simulink model "HevP1OptimalController"  (R2023b)
settings: configuration reference "VehicleFixed10ms" (kept outside this file)
model workspace (MAT data in the model file):
  N_P0 = 1
undefined symbols (not defined in the file): CtrlBcuTrlrBrkGain, CtrlVcuHevPxChrgLmtBpt, CtrlVcuHevPxRegenBrkCutOff, CtrlVcuHevPxSocBpt, PlntBrkActrBoreFrnt, PlntBrkFrntBias, PlntBrkKinFricCffFrnt, PlntBrkNumPadsFrnt, PlntBrkPadMeanRadiusFrnt, PlntBrkPrsFctr, PlntBrkRearBias, PlntDCDCEff, PlntDiffrntlEff, PlntDiffrntlRatio, PlntEM1EffTbl, PlntEM1Spd, PlntEM1Trq, PlntEngAccPwrTbl, PlntEngAccSpdBpt, PlntEngBrkTrqSpdBpt, PlntTransEffSpdBpt, PlntTransEffTbl, PlntTransEffTempBpt, PlntTransEffTrqBpt, PlntTransGearNumVect, PlntTransGearRatioVect, PlntWhlLdRadius
libraries: simulink x2, autolibhevctrlr x1, autolibhevctrlrcommon x1
settings Model: DataDictionary=VirtualVehicleTemplate.sldd  ModifiedByFormat=The MathWorks, Inc.  Creator=The MathWorks, Inc.  LastModifiedBy=The MathWorks, Inc.
settings ConfigSetRef: SourceName=VehicleFixed10ms

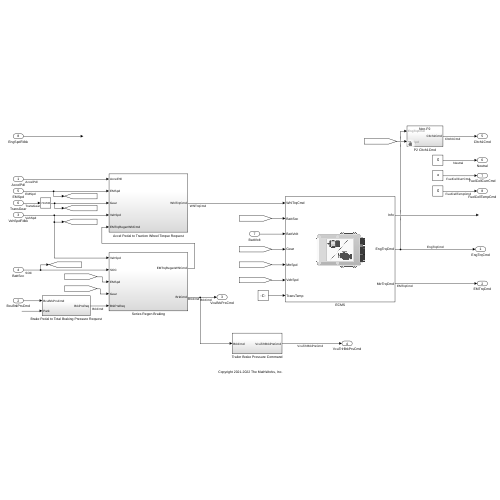
[thumbnail: Simulink's stored preview of the top-level diagram]
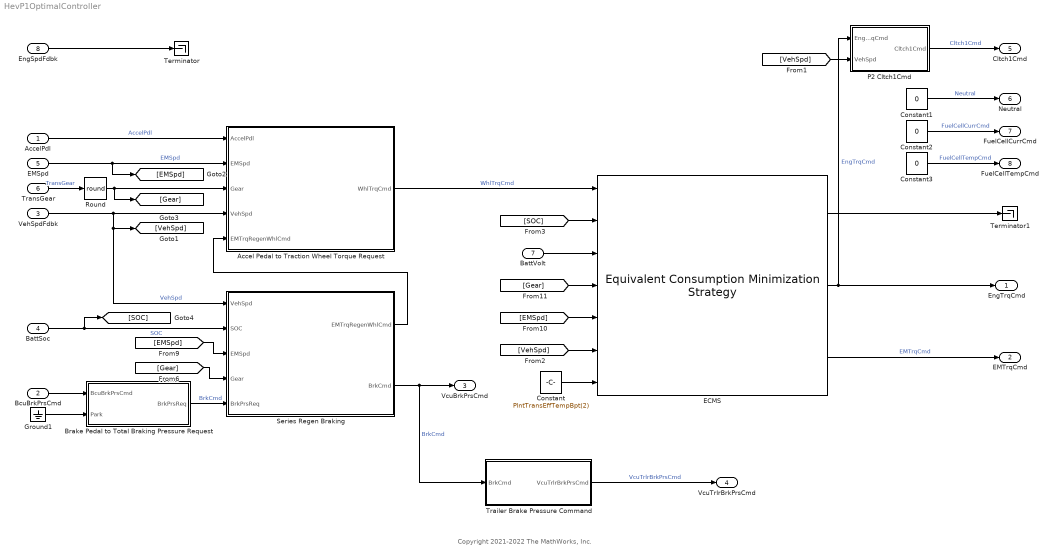
== system HevP1OptimalController ==
  note: Copyright 2021-2022 The MathWorks, Inc.
  AccelPdl : Inport  OutDataTypeStr=double  PortDimensions=1
  "   BcuBrkPrsCmd   " : Inport  Port=2  OutDataTypeStr=double  PortDimensions=4
  VehSpdFdbk : Inport  Port=3  OutDataTypeStr=double  PortDimensions=1
  BattSoc : Inport  Port=4  OutDataTypeStr=double  PortDimensions=1
  EMSpd : Inport  Port=5  OutDataTypeStr=double  PortDimensions=1
  TransGear : Inport  Port=6  OutDataTypeStr=double  PortDimensions=1
  BattVolt : Inport  Port=7  OutDataTypeStr=double  PortDimensions=1
  EngSpdFdbk : Inport  Port=8  OutDataTypeStr=double  PortDimensions=1
  Accel Pedal to Traction Wheel Torque Request : Subsystem  InitFcn=[~]=autosharedicon('autolibinternalvvblock',gcb,0);
  Brake Pedal to Total Braking Pressure Request : Subsystem
  Constant : Constant  Value=PlntTransEffTempBpt(2)
  Constant1 : Constant  Value=0  SampleTime=-1
  Constant2 : Constant  Value=0  SampleTime=-1
  Constant3 : Constant  Value=0  SampleTime=-1
  ECMS : autolibhevctrlr/Equivalent Consumption Minimization Strategy  HevMtrLoc=P1  EcmsMethod=Non-adaptive  N_diff=PlntDiffrntlRatio  eta_diff=PlntDiffrntlEff  N_diff_P4=PlntDiffrntl2Ratio  Re=PlntWhlLdRadius  TransEffFactors=Gear, input torque, input speed, and temperature  G_trans=PlntTransGearNumVect  N_trans=PlntTransGearRatioVect  Trq_trans_bpts=PlntTransEffTrqBpt  omega_trans_bpts=PlntTransEffSpdBpt  Temp_trans_bpts=PlntTransEffTempBpt  eta_trans=PlntTransEffVect  eta_trans_tbl=PlntTransEffTbl  f_tbrake_n_bpt=PlntEngBrkTrqSpdBpt  f_tbrake_t_bpt=PlntEngBrkTrqBpt  f_tbrake=PlntEngBrkTrqMap  f_tbrake_min=CtrlVcuHevPxEngTrqMin  f_fuel=PlntEngFuelFlwMap  HEVEngTrq_min=CtrlVcuHevPxHEVEngTrqMin  LHV=PlntEngLhv  AccPwrTbl=[0 0]  AccSpdBpts=[300 750]  N_idle=CtrlEcuNidle  SOC_bpt=CtrlVcuHevPxSocBpt  ChrgLmt=CtrlVcuHevPxChrgLmtBpt  DischrgLmt=CtrlVcuHevPxDischrgLmtBpt  BattCurrMax=CtrlVcuHevPxBattCurrMax  eta_dcdc=PlntDCDCEff/100  BattChrgPwrMax=CtrlVcuHevPxBattChrgPwrMax  BattDischrgPwrMax=CtrlVcuHevPxBattDischrgPwrMax  MtrEffiMethod=Positive speed and full torque range  f_tmtr_max=PlntEM1Trq  f_mtr_w_bpt=PlntEM1Spd*30/pi  f_mtr_t_bpt=PlntEM1TrqEff  f_mtr_eta=PlntEM1EffTbl/100  Ngrid=CtrlVcuHevPxNgrid  N_P0=PlntDiffrntlP0Ratio  ECMS_s=CtrlVcuHevP1ECMSs  a=CtrlVcuHevPxPnltyFctr  ECMS_Kp=CtrlVcuHevPxAdaptECMSKpGain  ECMS_Ki=CtrlVcuHevPxAdaptECMSKiGain  PenaltyFctr=CtrlVcuHevPxPenaltyFctr  SOCTrgt=CtrlVcuHevPxSOCTrgt  SOCmin=CtrlVcuHevPxSOCmin  SOCmax=CtrlVcuHevPxSOCmax
  Ground1 : Ground
  P2 Cltch1Cmd : Subsystem  Variant=on  VariantControlMode=label  VariantControl=1  LabelModeActiveChoice=0
  Round : Rounding  Operator=round
  Series Regen Braking : Subsystem  InitFcn=[~]=autosharedicon('autolibinternalvvblock',gcb,0);  VariantControl=0
  Terminator : Terminator
  Terminator1 : Terminator
  Trailer Brake Pressure Command : Subsystem
  EngTrqCmd : Outport  OutDataTypeStr=double  Unit=N*m  PortDimensions=1  VectorParamsAs1DForOutWhenUnconnected=off
  EMTrqCmd : Outport  Port=2  OutDataTypeStr=double  Unit=N*m  PortDimensions=1  VectorParamsAs1DForOutWhenUnconnected=off
  VcuBrkPrsCmd : Outport  Port=3  OutDataTypeStr=double  PortDimensions=4  VectorParamsAs1DForOutWhenUnconnected=off
  VcuTrlrBrkPrsCmd : Outport  Port=4  PortDimensions=6  VectorParamsAs1DForOutWhenUnconnected=off
  Cltch1Cmd : Outport  Port=5  OutDataTypeStr=double  PortDimensions=1  VectorParamsAs1DForOutWhenUnconnected=off
  Neutral : Outport  Port=6  OutDataTypeStr=double  PortDimensions=1  VectorParamsAs1DForOutWhenUnconnected=off
  FuelCellCurrCmd : Outport  Port=7  OutDataTypeStr=double  PortDimensions=1
  FuelCellTempCmd : Outport  Port=8  OutDataTypeStr=double  PortDimensions=1
  wires:
  AccelPdl/1 -> Accel Pedal to Traction Wheel Torque Request/1(AccelPdl)  "AccelPdl"
  "   BcuBrkPrsCmd   "/1 -> Brake Pedal to Total Braking Pressure Request/1(BcuBrkPrsCmd)
  VehSpdFdbk/1 -> Series Regen Braking/1(VehSpd), [VehSpd], Accel Pedal to Traction Wheel Torque Request/4(VehSpd)  "VehSpd"
  [SOC] -> ECMS/2
  EMSpd/1 -> [EMSpd], Accel Pedal to Traction Wheel Torque Request/2(EMSpd)  "EMSpd"
  Accel Pedal to Traction Wheel Torque Request/1(WhlTrqCmd) -> ECMS/1  "WhlTrqCmd"
  Ground1/1 -> Brake Pedal to Total Braking Pressure Request/2(Park)
  TransGear/1 -> Round/1  "TransGear"
  Brake Pedal to Total Braking Pressure Request/1(BrkPrsReq) -> Series Regen Braking/5("BrkPrsReq ")  "BrkCmd"
  Series Regen Braking/1(" EMTrqRegenWhlCmd") -> Accel Pedal to Traction Wheel Torque Request/5(EMTrqRegenWhlCmd)
  [EMSpd] -> Series Regen Braking/3(EMSpd)
  [Gear] -> Series Regen Braking/4(Gear)
  Constant1/1 -> Neutral/1  "Neutral"
  [VehSpd] -> ECMS/6
  [EMSpd] -> ECMS/5
  Constant/1 -> ECMS/7
  [Gear] -> ECMS/4
  BattVolt/1 -> ECMS/3
  EngSpdFdbk/1 -> Terminator/1
  BattSoc/1 -> Series Regen Braking/2(SOC), [SOC]  "SOC"
  Round/1 -> [Gear], Accel Pedal to Traction Wheel Torque Request/3(Gear)
  ECMS/3 -> EMTrqCmd/1  "EMTrqCmd"
  ECMS/2 -> EngTrqCmd/1, P2 Cltch1Cmd/1(EngTrqCmd)  "EngTrqCmd"
  ECMS/1 -> Terminator1/1
  [VehSpd] -> P2 Cltch1Cmd/2(VehSpd)
  P2 Cltch1Cmd/1(Cltch1Cmd) -> Cltch1Cmd/1  "Cltch1Cmd"
  Constant2/1 -> FuelCellCurrCmd/1  "FuelCellCurrCmd"
  Constant3/1 -> FuelCellTempCmd/1  "FuelCellTempCmd"
  Series Regen Braking/2(" BrkCmd") -> Trailer Brake Pressure Command/1(BrkCmd), VcuBrkPrsCmd/1  "BrkCmd"
  Trailer Brake Pressure Command/1(VcuTrlrBrkPrsCmd) -> VcuTrlrBrkPrsCmd/1  "VcuTrlrBrkPrsCmd"

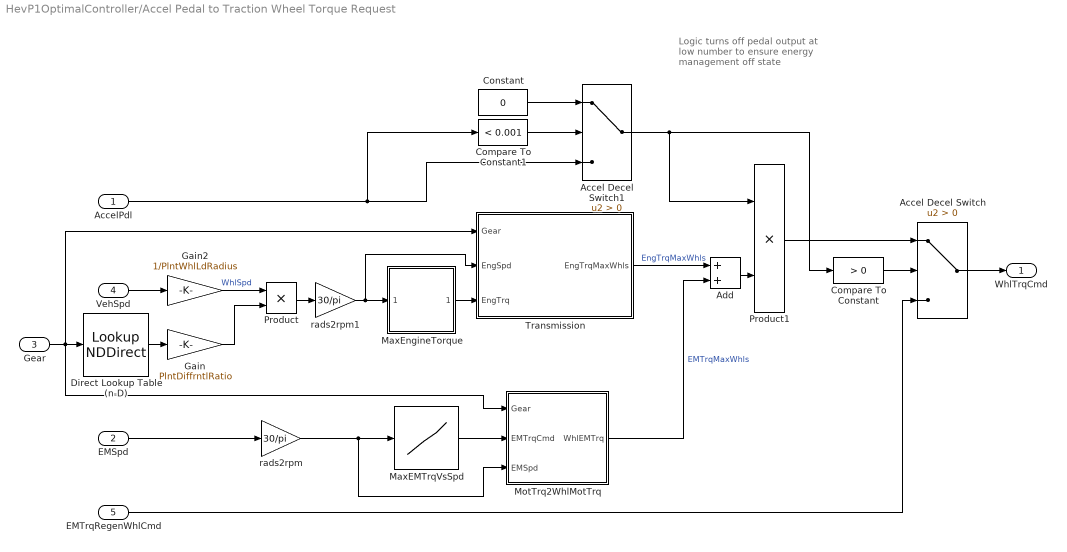
== system HevP1OptimalController/Accel Pedal to Traction Wheel Torque Request ==
  note: Logic turns off pedal
      | output at low number
      | to ensure energy
      | management off state
  AccelPdl : Inport
  EMSpd : Inport  Port=2
  Gear : Inport  Port=3
  VehSpd : Inport  Port=4
  EMTrqRegenWhlCmd : Inport  Port=5
  Accel Decel Switch : Switch  Criteria=u2 > Threshold  SaturateOnIntegerOverflow=off  InputSameDT=off
  Accel Decel Switch1 : Switch  Criteria=u2 > Threshold  SaturateOnIntegerOverflow=off  InputSameDT=off
  Add : Sum
  Compare To Constant : simulink/Logic and Bit Operations/Compare To Constant  relop=>  const=0  OutDataTypeStr=boolean
  Compare To Constant1 : simulink/Logic and Bit Operations/Compare To Constant  relop=<  const=0.001  OutDataTypeStr=boolean
  Constant : Constant  Value=0
  Direct Lookup Table (n-D) : LookupNDDirect  NumberOfTableDimensions=1  Table=PlntTransGearRatioVect
  Gain : Gain  Gain=PlntDiffrntlRatio
  Gain2 : Gain  Gain=1/PlntWhlLdRadius
  MaxEMTrqVsSpd : Lookup_n-D  NumberOfTableDimensions=1  BreakpointsForDimension1=PlntEM1Spd*30/pi  Table=PlntEM1Trq  ExtrapMethod=Clip  UseLastTableValue=on  InternalRulePriority=Speed  OutDataTypeStr=Inherit: Inherit from 'Table data'  RndMeth=Simplest
  MaxEngineTorque : Subsystem
  MotTrq2WhlMotTrq : Subsystem  VariantControl=1
  Product : Product
  Product1 : Product
  Transmission : Subsystem
  rads2rpm : Gain  Gain=30/pi
  rads2rpm1 : Gain  Gain=30/pi
  WhlTrqCmd : Outport  VectorParamsAs1DForOutWhenUnconnected=off
  wires:
  AccelPdl/1 -> Compare To Constant1/1, Accel Decel Switch1/3
  MaxEngineTorque/1(EngTrq) -> Transmission/3(EngTrq)
  MaxEMTrqVsSpd/1 -> MotTrq2WhlMotTrq/2(EMTrqCmd)
  rads2rpm/1 -> MotTrq2WhlMotTrq/3(EMSpd), MaxEMTrqVsSpd/1
  EMSpd/1 -> rads2rpm/1
  Gear/1 -> MotTrq2WhlMotTrq/1(Gear), Transmission/1(Gear), Direct Lookup Table (n-D)/1
  EMTrqRegenWhlCmd/1 -> Accel Decel Switch/3
  Compare To Constant/1 -> Accel Decel Switch/2
  Product1/1 -> Accel Decel Switch/1
  Accel Decel Switch/1 -> WhlTrqCmd/1
  MotTrq2WhlMotTrq/1(WhlEMTrq) -> Add/2  "EMTrqMaxWhls"
  VehSpd/1 -> Gain2/1
  Gain2/1 -> Product/1  "WhlSpd"
  Gain/1 -> Product/2
  Product/1 -> rads2rpm1/1
  rads2rpm1/1 -> MaxEngineTorque/1(EngSpd), Transmission/2(EngSpd)
  Direct Lookup Table (n-D)/1 -> Gain/1
  Transmission/1(EngTrqMaxWhls) -> Add/1  "EngTrqMaxWhls"
  Add/1 -> Product1/2
  Compare To Constant1/1 -> Accel Decel Switch1/2
  Accel Decel Switch1/1 -> Product1/1, Compare To Constant/1
  Constant/1 -> Accel Decel Switch1/1

== system HevP1OptimalController/Brake Pedal to Total Braking Pressure Request ==
  BcuBrkPrsCmd : Inport
  Park : Inport  Port=2
  Front Bias : Constant  Value=PlntBrkFrntBias
  Gain4 : Gain  Gain=PlntBrkPrsFctr
  Mux : Mux
  Product : Product
  Rear Bias : Constant  Value=PlntBrkRearBias
  Terminator : Terminator
  BrkPrsReq : Outport  VectorParamsAs1DForOutWhenUnconnected=off
  wires:
  BcuBrkPrsCmd/1 -> Product/2
  Mux/1 -> Product/1
  Rear Bias/1 -> Mux/4, Mux/3
  Front Bias/1 -> Mux/1, Mux/2
  Gain4/1 -> BrkPrsReq/1
  Product/1 -> Gain4/1
  Park/1 -> Terminator/1

== system HevP1OptimalController/P2 Cltch1Cmd ==
  EngTrqCmd : Inport
  VehSpd : Inport  Port=2
  Non-P2 : Subsystem  VariantControl=0
  P2 Cltch1Cmd : Subsystem  VariantControl=1
  Cltch1Cmd : Outport

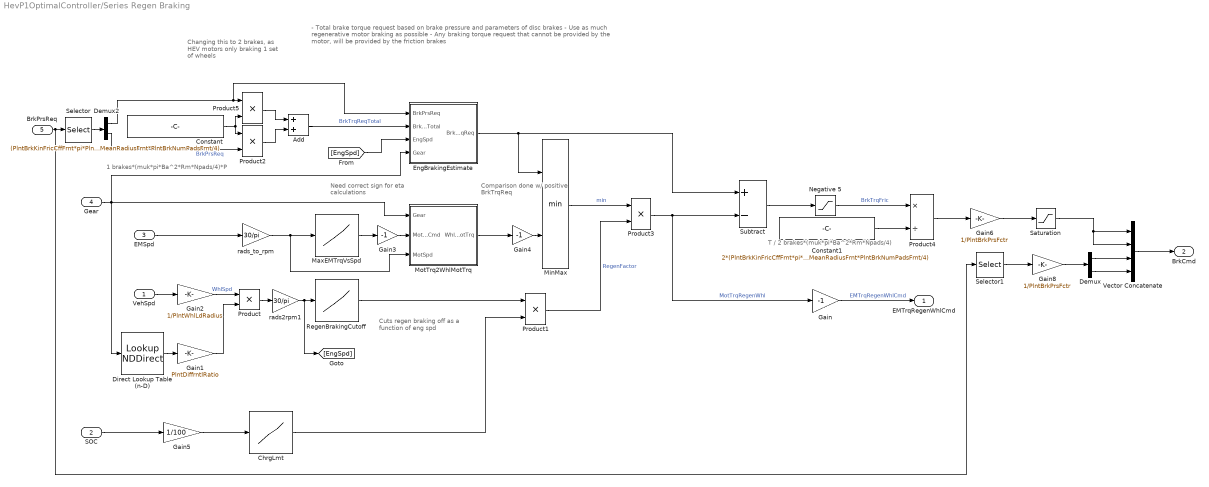
== system HevP1OptimalController/Series Regen Braking ==
  note: Changing this to 2 brakes,
      | as HEV motors only braking
      | 1 set of wheels
  note: Comparison done
      | w/ positive BrkTrqReq
  note: Need correct sign
      | for eta calculations
  note: Cuts regen braking off
      | as a function of eng spd
  note: - Total brake torque request based on brake pressure and parameters of disc brakes
      | - Use as much regenerative motor braking as possible
      | -  Any braking torque request that cannot be provided by the motor, will be provided by the friction brakes
  note: T / 2 brakes*(muk*pi*Ba^2*Rm*Npads/4)
  note: 1 brakes*(muk*pi*Ba^2*Rm*Npads/4)*P
  VehSpd : Inport
  SOC : Inport  Port=2
  EMSpd : Inport  Port=3
  Gear : Inport  Port=4
  "BrkPrsReq " : Inport  Port=5
  Add : Sum
  ChrgLmt : Lookup_n-D  NumberOfTableDimensions=1  BreakpointsForDimension1=CtrlVcuHevPxSocBpt  Table=CtrlVcuHevPxChrgLmtBpt  ExtrapMethod=Clip  UseLastTableValue=on  InternalRulePriority=Speed  RndMeth=Simplest
  Constant : Constant  Value=(PlntBrkKinFricCffFrnt*pi*PlntBrkActrBoreFrnt^2*PlntBrkPadMeanRadiusFrnt*PlntBrkNumPadsFrnt/4)
  Constant1 : Constant  Value=2*(PlntBrkKinFricCffFrnt*pi*PlntBrkActrBoreFrnt^2*PlntBrkPadMeanRadiusFrnt*PlntBrkNumPadsFrnt/4)
  Demux : Demux  Outputs=2
  Demux2 : Demux  Outputs=2
  Direct Lookup Table (n-D) : LookupNDDirect  NumberOfTableDimensions=1  Table=PlntTransGearRatioVect
  EngBrakingEstimate : Subsystem
  Gain : Gain  Gain=-1
  Gain1 : Gain  Gain=PlntDiffrntlRatio
  Gain2 : Gain  Gain=1/PlntWhlLdRadius
  Gain3 : Gain  Gain=-1
  Gain4 : Gain  Gain=-1
  Gain5 : Gain  Gain=1/100
  Gain6 : Gain  Gain=1/PlntBrkPrsFctr
  Gain8 : Gain  Gain=1/PlntBrkPrsFctr
  MaxEMTrqVsSpd : Lookup_n-D  NumberOfTableDimensions=1  BreakpointsForDimension1=PlntEM1Spd*30/pi  Table=PlntEM1Trq  ExtrapMethod=Clip  UseLastTableValue=on  InternalRulePriority=Speed  OutDataTypeStr=Inherit: Inherit from 'Table data'  RndMeth=Simplest
  MinMax : MinMax  Inputs=2
  MotTrq2WhlMotTrq : Subsystem  VariantControl=1
  Negative 5 : Saturate  UpperLimit=inf  LowerLimit=0
  Product{,1..3,5} (5 alike) : Product
  Product4 : Product  Inputs=*/
  RegenBrakingCutoff : Lookup_n-D  NumberOfTableDimensions=1  BreakpointsForDimension1=[PlntEngBrkTrqSpdBpt(2) PlntEngBrkTrqSpdBpt(3)]  Table=CtrlVcuHevPxRegenBrkCutOff  ExtrapMethod=Clip  UseLastTableValue=on  InternalRulePriority=Speed  RndMeth=Simplest
  Saturation : Saturate  UpperLimit=1  LowerLimit=0
  Selector : Selector  InputPortWidth=4  IndexOptions=Index vector (dialog)  Indices=[1 2]  OutputSizes=1
  Selector1 : Selector  InputPortWidth=4  IndexOptions=Index vector (dialog)  Indices=[3 4]  OutputSizes=1
  Subtract : Sum  Inputs=+-
  Vector Concatenate : Concatenate  NumInputs=4
  rads2rpm1 : Gain  Gain=30/pi
  rads_to_rpm : Gain  Gain=30/pi
  " EMTrqRegenWhlCmd" : Outport  VectorParamsAs1DForOutWhenUnconnected=off
  " BrkCmd" : Outport  Port=2  VectorParamsAs1DForOutWhenUnconnected=off
  wires:
  Product3/1 -> Gain/1, Subtract/2  "MotTrqRegenWhl"
  Constant1/1 -> Product4/2
  Constant/1 -> Product5/2, Product2/1
  Demux2/2 -> Product2/2  "BrkPrsReq"
  rads_to_rpm/1 -> MotTrq2WhlMotTrq/3(MotSpd), MaxEMTrqVsSpd/1
  Gain3/1 -> MotTrq2WhlMotTrq/2(MotTrqCmd)
  MinMax/1 -> Product3/1  "min"
  RegenBrakingCutoff/1 -> Product1/1
  Subtract/1 -> Negative 5/1
  Negative 5/1 -> Product4/1  "BrkTrqFric"
  EMSpd/1 -> rads_to_rpm/1
  MotTrq2WhlMotTrq/1(WhlMotTrq) -> Gain4/1
  Gain/1 -> " EMTrqRegenWhlCmd"/1  "EMTrqRegenWhlCmd"
  Gear/1 -> MotTrq2WhlMotTrq/1(Gear), Direct Lookup Table (n-D)/1, EngBrakingEstimate/4(Gear)
  Gain1/1 -> Product/2
  Product/1 -> rads2rpm1/1
  Direct Lookup Table (n-D)/1 -> Gain1/1
  VehSpd/1 -> Gain2/1
  Gain2/1 -> Product/1  "WhlSpd"
  rads2rpm1/1 -> [EngSpd], RegenBrakingCutoff/1
  MaxEMTrqVsSpd/1 -> Gain3/1
  Gain4/1 -> MinMax/2
  EngBrakingEstimate/1(BrkTrqReq) -> Subtract/1, MinMax/1
  Add/1 -> EngBrakingEstimate/2(BrkTrqReqTotal)  "BrkTrqReqTotal"
  [EngSpd] -> EngBrakingEstimate/3(EngSpd)
  SOC/1 -> Gain5/1
  Gain5/1 -> ChrgLmt/1
  ChrgLmt/1 -> Product1/2
  Product1/1 -> Product3/2  "RegenFactor"
  "BrkPrsReq "/1 -> Selector1/1, Selector/1
  Selector/1 -> Demux2/1
  Demux2/1 -> EngBrakingEstimate/1(BrkPrsReq), Product5/1
  Product4/1 -> Gain6/1
  Gain6/1 -> Saturation/1
  Selector1/1 -> Gain8/1
  Demux/2 -> Vector Concatenate/4
  Demux/1 -> Vector Concatenate/3
  Vector Concatenate/1 -> " BrkCmd"/1
  Saturation/1 -> Vector Concatenate/2, Vector Concatenate/1
  Gain8/1 -> Demux/1
  Product5/1 -> Add/1
  Product2/1 -> Add/2

== system HevP1OptimalController/Trailer Brake Pressure Command ==
  BrkCmd : Inport
  Gain1 : Gain  Gain=CtrlBcuTrlrBrkGain
  Probe : Probe  ProbeSampleTime=off  ProbeComplexSignal=off
  Product : Product  Inputs=*/
  Selector2 : Selector  InputPortWidth=1  IndexOptions=Index vector (dialog)  Indices=[1 1 1 1 1 1]  OutputSizes=1
  Sum : Sum  Inputs=+
  VcuTrlrBrkPrsCmd : Outport
  wires:
  Gain1/1 -> Selector2/1
  Product/1 -> Gain1/1
  Probe/1 -> Product/2
  BrkCmd/1 -> Probe/1, Sum/1
  Sum/1 -> Product/1
  Selector2/1 -> VcuTrlrBrkPrsCmd/1

== system HevP1OptimalController/Accel Pedal to Traction Wheel Torque Request/MaxEngineTorque ==
  note: Account for net torque of
      | eng due to accessory load
  EngSpd : Inport
  Accessory Load Model : Subsystem
  MaxEngineTorque : Lookup_n-D  NumberOfTableDimensions=1  BreakpointsForDimension1=PlntEngBrkTrqSpdBpt  Table=[0 max(PlntEngBrkTrqMap(:,2:end))]  ExtrapMethod=Clip  UseLastTableValue=on  InternalRulePriority=Speed  RndMeth=Simplest
  Minus : Sum  Inputs=+-
  EngTrq : Outport
  wires:
  EngSpd/1 -> MaxEngineTorque/1, Accessory Load Model/1(Engine Speed)
  Minus/1 -> EngTrq/1
  Accessory Load Model/1(Accessory Torque) -> Minus/2
  MaxEngineTorque/1 -> Minus/1

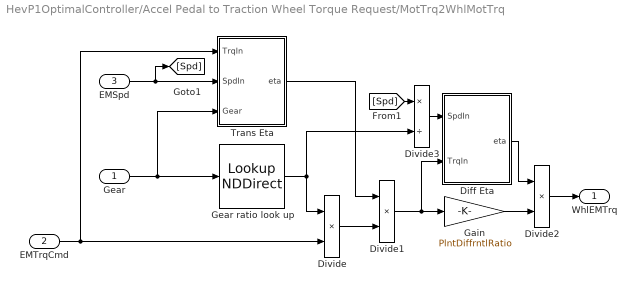
== system HevP1OptimalController/Accel Pedal to Traction Wheel Torque Request/MotTrq2WhlMotTrq ==
  Gear : Inport
  EMTrqCmd : Inport  Port=2
  EMSpd : Inport  Port=3
  Diff Eta : Subsystem
  Divide : Product  Inputs=**
  Divide1 : Product  Inputs=**
  Divide2 : Product  Inputs=**
  Divide3 : Product  Inputs=*/
  Gain : Gain  Gain=PlntDiffrntlRatio
  Gear ratio look up : LookupNDDirect  NumberOfTableDimensions=1  Table=PlntTransGearRatioVect
  Trans Eta : Subsystem
  WhlEMTrq : Outport  VectorParamsAs1DForOutWhenUnconnected=off
  wires:
  Gain/1 -> Divide2/2
  Gear ratio look up/1 -> Divide3/2, Divide/1
  Divide/1 -> Divide1/2
  Gear/1 -> Trans Eta/3(Gear), Gear ratio look up/1
  Trans Eta/1(eta) -> Divide1/1
  Divide1/1 -> Diff Eta/2(TrqIn), Gain/1
  EMTrqCmd/1 -> Trans Eta/1(TrqIn), Divide/2
  EMSpd/1 -> [Spd], Trans Eta/2(SpdIn)
  Divide2/1 -> WhlEMTrq/1
  Diff Eta/1(eta) -> Divide2/1
  [Spd] -> Divide3/1
  Divide3/1 -> Diff Eta/1(SpdIn)

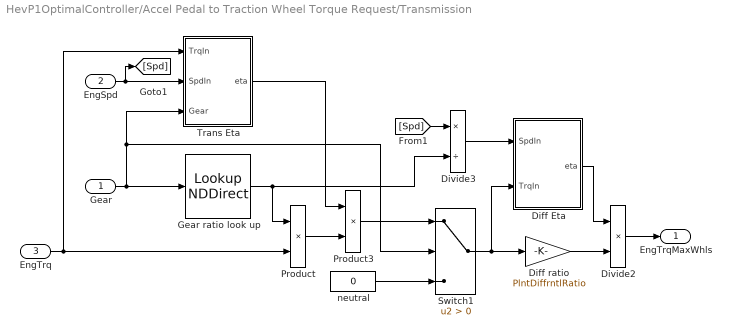
== system HevP1OptimalController/Accel Pedal to Traction Wheel Torque Request/Transmission ==
  Gear : Inport
  EngSpd : Inport  Port=2
  EngTrq : Inport  Port=3
  Diff Eta : Subsystem
  Diff ratio : Gain  Gain=PlntDiffrntlRatio
  Divide2 : Product  Inputs=**
  Divide3 : Product  Inputs=*/
  Gear ratio look up : LookupNDDirect  NumberOfTableDimensions=1  Table=PlntTransGearRatioVect
  Product : Product  RndMeth=Zero
  Product3 : Product  Inputs=**  RndMeth=Zero
  Switch1 : Switch  Criteria=u2 > Threshold  SaturateOnIntegerOverflow=off  InputSameDT=off
  Trans Eta : Subsystem
  neutral : Constant  Value=0
  EngTrqMaxWhls : Outport  VectorParamsAs1DForOutWhenUnconnected=off
  wires:
  Product/1 -> Product3/2
  Switch1/1 -> Diff Eta/2(TrqIn), Diff ratio/1
  Gear ratio look up/1 -> Divide3/2, Product/1
  Gear/1 -> Gear ratio look up/1, Trans Eta/3(Gear), Switch1/2
  Trans Eta/1(eta) -> Product3/1
  neutral/1 -> Switch1/3
  Product3/1 -> Switch1/1
  Diff ratio/1 -> Divide2/2
  EngSpd/1 -> [Spd], Trans Eta/2(SpdIn)
  EngTrq/1 -> Trans Eta/1(TrqIn), Product/2
  Diff Eta/1(eta) -> Divide2/1
  Divide2/1 -> EngTrqMaxWhls/1
  Divide3/1 -> Diff Eta/1(SpdIn)
  [Spd] -> Divide3/1

== system HevP1OptimalController/P2 Cltch1Cmd/Non-P2 ==
  Constant : Constant  Value=0  SampleTime=-1
  Cltch1Cmd : Outport  VectorParamsAs1DForOutWhenUnconnected=off
  wires:
  Constant/1 -> Cltch1Cmd/1  "Cltch1Cmd"

== system HevP1OptimalController/P2 Cltch1Cmd/P2 Cltch1Cmd ==
  EngTrqCmd : Inport
  VehSpd : Inport  Port=2
  Chart : Stateflow chart  TreatAsAtomicUnit=on
  Cltch1Cmd : Outport  VectorParamsAs1DForOutWhenUnconnected=off
  wires:
  Chart/1(Cltch1Cmd) -> Cltch1Cmd/1  "Cltch1Cmd"
  EngTrqCmd/1 -> Chart/1(EngTrqCmd)
  VehSpd/1 -> Chart/2(VehSpd)

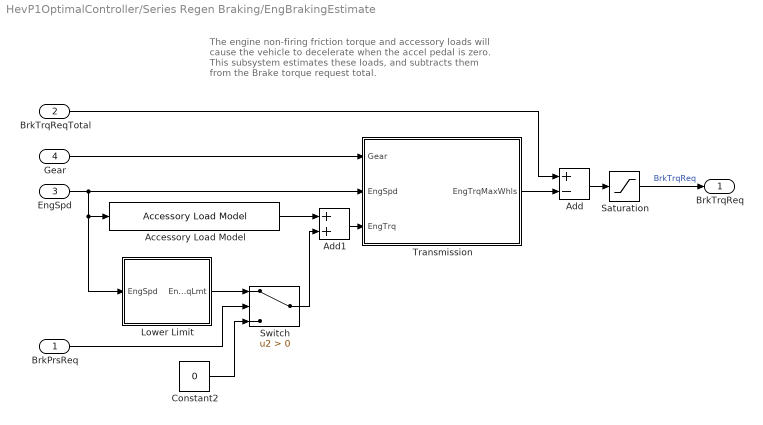
== system HevP1OptimalController/Series Regen Braking/EngBrakingEstimate ==
  note: The engine non-firing friction torque and accessory loads
      | will cause the vehicle to decelerate when the accel pedal
      | is zero.  This subsystem estimates these loads, and
      | subtracts them from the Brake torque request total.
  BrkPrsReq : Inport
  BrkTrqReqTotal : Inport  Port=2
  EngSpd : Inport  Port=3
  Gear : Inport  Port=4
  Accessory Load Model : autolibhevctrlrcommon/Accessory Load Model  AccPwrTbl=[0 0]  AccSpdBpts=[300 750]
  Add : Sum  Inputs=+-
  Add1 : Sum
  Constant2 : Constant  Value=0
  Lower Limit : Subsystem
  Saturation : Saturate  UpperLimit=inf  LowerLimit=0
  Switch : Switch  Criteria=u2 > Threshold  SaturateOnIntegerOverflow=off  InputSameDT=off
  Transmission : Subsystem
  BrkTrqReq : Outport  VectorParamsAs1DForOutWhenUnconnected=off
  wires:
  EngSpd/1 -> Lower Limit/1(EngSpd), Accessory Load Model/1, Transmission/2(EngSpd)
  Add/1 -> Saturation/1
  Switch/1 -> Add1/2
  Saturation/1 -> BrkTrqReq/1  "BrkTrqReq"
  Lower Limit/1(EngTrqLmt) -> Switch/1
  BrkTrqReqTotal/1 -> Add/1
  Accessory Load Model/1 -> Add1/1
  Constant2/1 -> Switch/3
  Add1/1 -> Transmission/3(EngTrq)
  Transmission/1(EngTrqMaxWhls) -> Add/2
  BrkPrsReq/1 -> Switch/2
  Gear/1 -> Transmission/1(Gear)

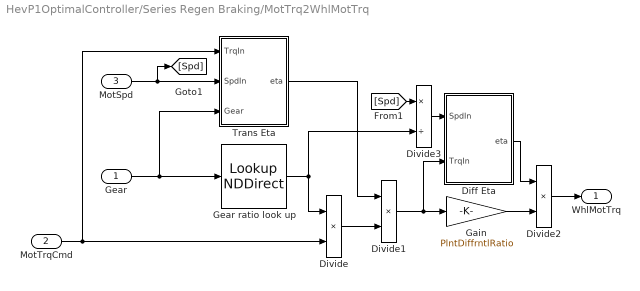
== system HevP1OptimalController/Series Regen Braking/MotTrq2WhlMotTrq ==
  Gear : Inport
  MotTrqCmd : Inport  Port=2
  MotSpd : Inport  Port=3
  Diff Eta : Subsystem
  Divide : Product  Inputs=**
  Divide1 : Product  Inputs=**
  Divide2 : Product  Inputs=**
  Divide3 : Product  Inputs=*/
  Gain : Gain  Gain=PlntDiffrntlRatio
  Gear ratio look up : LookupNDDirect  NumberOfTableDimensions=1  Table=PlntTransGearRatioVect
  Trans Eta : Subsystem
  WhlMotTrq : Outport  VectorParamsAs1DForOutWhenUnconnected=off
  wires:
  Gain/1 -> Divide2/2
  Gear ratio look up/1 -> Divide3/2, Divide/1
  Divide/1 -> Divide1/2
  Gear/1 -> Trans Eta/3(Gear), Gear ratio look up/1
  Trans Eta/1(eta) -> Divide1/1
  Divide1/1 -> Diff Eta/2(TrqIn), Gain/1
  MotTrqCmd/1 -> Trans Eta/1(TrqIn), Divide/2
  MotSpd/1 -> [Spd], Trans Eta/2(SpdIn)
  Divide2/1 -> WhlMotTrq/1
  Diff Eta/1(eta) -> Divide2/1
  [Spd] -> Divide3/1
  Divide3/1 -> Diff Eta/1(SpdIn)

== system HevP1OptimalController/Accel Pedal to Traction Wheel Torque Request/MaxEngineTorque/Accessory Load Model ==
  Engine Speed : Inport
  Accessory Load Power : Lookup_n-D  NumberOfTableDimensions=1  LookupTableObject=''  BreakpointsForDimension1=PlntEngAccSpdBpt  Table=PlntEngAccPwrTbl  ExtrapMethod=Clip  InternalRulePriority=Speed  RndMeth=Simplest
  Divide : Product  Inputs=*/
  Kw to w : Gain  Gain=1000
  Saturation : Saturate  UpperLimit=Inf  LowerLimit=300
  rpm to rad/s : Gain  Gain=pi/30
  Accessory Torque : Outport  VectorParamsAs1DForOutWhenUnconnected=off
  wires:
  Divide/1 -> Accessory Torque/1
  Accessory Load Power/1 -> Kw to w/1
  Engine Speed/1 -> Accessory Load Power/1, Saturation/1
  Saturation/1 -> rpm to rad/s/1
  rpm to rad/s/1 -> Divide/2
  Kw to w/1 -> Divide/1

== system HevP1OptimalController/Accel Pedal to Traction Wheel Torque Request/MotTrq2WhlMotTrq/Diff Eta ==
  SpdIn : Inport
  TrqIn : Inport  Port=2
  Constant : Constant  Value=PlntDiffrntlEff
  Constant1 : Constant  SampleTime=-1
  Constant2 : Constant  Value=-1  SampleTime=-1
  Math Function1 : Math  Operator=pow  SignedPower=on  OutputSignalType=real
  Product1 : Product
  Switch2 : Switch  SaturateOnIntegerOverflow=off  InputSameDT=off
  rpm2rads : Gain  Gain=pi/30
  eta : Outport  VectorParamsAs1DForOutWhenUnconnected=off
  wires:
  rpm2rads/1 -> Product1/2
  Constant/1 -> Math Function1/1
  Constant2/1 -> Switch2/3
  Constant1/1 -> Switch2/1
  Product1/1 -> Switch2/2
  Switch2/1 -> Math Function1/2
  Math Function1/1 -> eta/1
  SpdIn/1 -> rpm2rads/1
  TrqIn/1 -> Product1/1

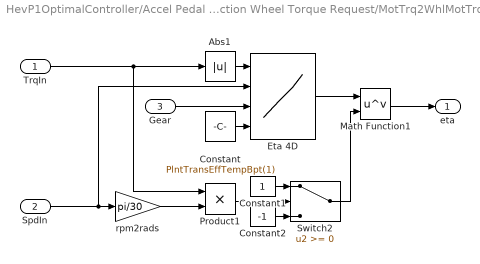
== system HevP1OptimalController/Accel Pedal to Traction Wheel Torque Request/MotTrq2WhlMotTrq/Trans Eta ==
  TrqIn : Inport
  SpdIn : Inport  Port=2
  Gear : Inport  Port=3
  Abs1 : Abs  SaturateOnIntegerOverflow=off
  Constant : Constant  Value=PlntTransEffTempBpt(1)
  Constant1 : Constant  SampleTime=-1
  Constant2 : Constant  Value=-1  SampleTime=-1
  Eta 4D : Lookup_n-D  NumberOfTableDimensions=4  LookupTableObject=''  BreakpointsForDimension1=PlntTransEffTrqBpt  BreakpointsForDimension2=PlntTransEffSpdBpt  BreakpointsForDimension3=PlntTransGearNumVect  BreakpointsForDimension4=PlntTransEffTempBpt  Table=PlntTransEffTbl  ExtrapMethod=Clip  InternalRulePriority=Speed  RndMeth=Simplest
      settings: InputPortMap=u0,u1,u2,u3
  Math Function1 : Math  Operator=pow  SignedPower=on  OutputSignalType=real
  Product1 : Product
  Switch2 : Switch  SaturateOnIntegerOverflow=off  InputSameDT=off
  rpm2rads : Gain  Gain=pi/30
  eta : Outport  VectorParamsAs1DForOutWhenUnconnected=off
  wires:
  TrqIn/1 -> Product1/1, Abs1/1
  SpdIn/1 -> Eta 4D/2, rpm2rads/1
  Math Function1/1 -> eta/1
  Abs1/1 -> Eta 4D/1
  Switch2/1 -> Math Function1/2
  Product1/1 -> Switch2/2
  Constant1/1 -> Switch2/1
  Constant2/1 -> Switch2/3
  Eta 4D/1 -> Math Function1/1
  rpm2rads/1 -> Product1/2
  Gear/1 -> Eta 4D/3
  Constant/1 -> Eta 4D/4

== system HevP1OptimalController/Accel Pedal to Traction Wheel Torque Request/Transmission/Diff Eta ==
  SpdIn : Inport
  TrqIn : Inport  Port=2
  Constant : Constant  Value=PlntDiffrntlEff
  Constant1 : Constant  SampleTime=-1
  Constant2 : Constant  Value=-1  SampleTime=-1
  Math Function1 : Math  Operator=pow  SignedPower=on  OutputSignalType=real
  Product1 : Product
  Switch2 : Switch  SaturateOnIntegerOverflow=off  InputSameDT=off
  rpm2rads : Gain  Gain=pi/30
  eta : Outport  VectorParamsAs1DForOutWhenUnconnected=off
  wires:
  rpm2rads/1 -> Product1/2
  Constant/1 -> Math Function1/1
  Constant2/1 -> Switch2/3
  Constant1/1 -> Switch2/1
  Product1/1 -> Switch2/2
  Switch2/1 -> Math Function1/2
  Math Function1/1 -> eta/1
  SpdIn/1 -> rpm2rads/1
  TrqIn/1 -> Product1/1

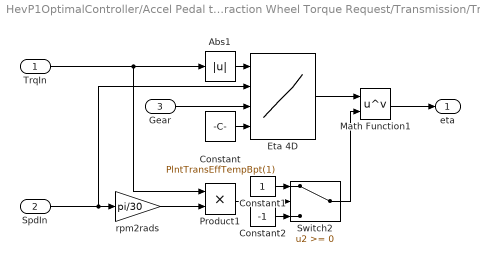
== system HevP1OptimalController/Accel Pedal to Traction Wheel Torque Request/Transmission/Trans Eta ==
  TrqIn : Inport
  SpdIn : Inport  Port=2
  Gear : Inport  Port=3
  Abs1 : Abs  SaturateOnIntegerOverflow=off
  Constant : Constant  Value=PlntTransEffTempBpt(1)
  Constant1 : Constant  SampleTime=-1
  Constant2 : Constant  Value=-1  SampleTime=-1
  Eta 4D : Lookup_n-D  NumberOfTableDimensions=4  LookupTableObject=''  BreakpointsForDimension1=PlntTransEffTrqBpt  BreakpointsForDimension2=PlntTransEffSpdBpt  BreakpointsForDimension3=PlntTransGearNumVect  BreakpointsForDimension4=PlntTransEffTempBpt  Table=PlntTransEffTbl  ExtrapMethod=Clip  InternalRulePriority=Speed  RndMeth=Simplest
      settings: InputPortMap=u0,u1,u2,u3
  Math Function1 : Math  Operator=pow  SignedPower=on  OutputSignalType=real
  Product1 : Product
  Switch2 : Switch  SaturateOnIntegerOverflow=off  InputSameDT=off
  rpm2rads : Gain  Gain=pi/30
  eta : Outport  VectorParamsAs1DForOutWhenUnconnected=off
  wires:
  TrqIn/1 -> Product1/1, Abs1/1
  SpdIn/1 -> Eta 4D/2, rpm2rads/1
  Math Function1/1 -> eta/1
  Abs1/1 -> Eta 4D/1
  Switch2/1 -> Math Function1/2
  Product1/1 -> Switch2/2
  Constant1/1 -> Switch2/1
  Constant2/1 -> Switch2/3
  Eta 4D/1 -> Math Function1/1
  rpm2rads/1 -> Product1/2
  Gear/1 -> Eta 4D/3
  Constant/1 -> Eta 4D/4

== system HevP1OptimalController/Series Regen Braking/EngBrakingEstimate/Lower Limit ==
  note: Engine non-firing friction torque
      | (0 torque command row of f_tbrake map)
  EngSpd : Inport
  Gain5 : Gain  Gain=-1
  Max Torque vs Speed : Lookup_n-D  NumberOfTableDimensions=1  BreakpointsForDimension1=[0 749 PlntEngBrkTrqSpdBpt(:,2:end)]  Table=[0 0 min(PlntEngBrkTrqMap(:,2:end))]  ExtrapMethod=Clip  UseLastTableValue=on  RndMeth=Simplest
  Saturation1 : Saturate  UpperLimit=inf  LowerLimit=0
  EngTrqLmt : Outport  VectorParamsAs1DForOutWhenUnconnected=off
  wires:
  EngSpd/1 -> Max Torque vs Speed/1
  Gain5/1 -> Saturation1/1
  Max Torque vs Speed/1 -> Gain5/1
  Saturation1/1 -> EngTrqLmt/1

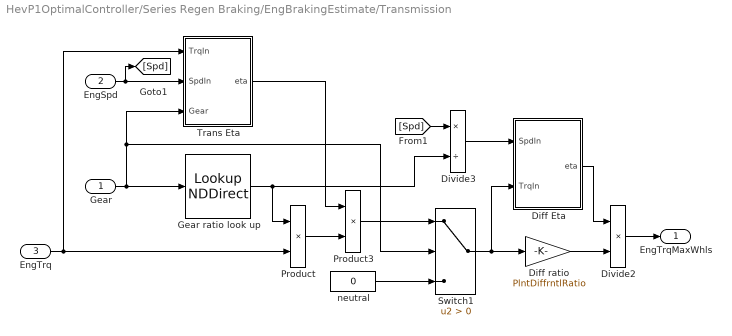
== system HevP1OptimalController/Series Regen Braking/EngBrakingEstimate/Transmission ==
  Gear : Inport
  EngSpd : Inport  Port=2
  EngTrq : Inport  Port=3
  Diff Eta : Subsystem
  Diff ratio : Gain  Gain=PlntDiffrntlRatio
  Divide2 : Product  Inputs=**
  Divide3 : Product  Inputs=*/
  Gear ratio look up : LookupNDDirect  NumberOfTableDimensions=1  Table=PlntTransGearRatioVect
  Product : Product  RndMeth=Zero
  Product3 : Product  Inputs=**  RndMeth=Zero
  Switch1 : Switch  Criteria=u2 > Threshold  SaturateOnIntegerOverflow=off  InputSameDT=off
  Trans Eta : Subsystem
  neutral : Constant  Value=0
  EngTrqMaxWhls : Outport  VectorParamsAs1DForOutWhenUnconnected=off
  wires:
  Product/1 -> Product3/2
  Switch1/1 -> Diff Eta/2(TrqIn), Diff ratio/1
  Gear ratio look up/1 -> Divide3/2, Product/1
  Gear/1 -> Gear ratio look up/1, Trans Eta/3(Gear), Switch1/2
  Trans Eta/1(eta) -> Product3/1
  neutral/1 -> Switch1/3
  Product3/1 -> Switch1/1
  Diff ratio/1 -> Divide2/2
  EngSpd/1 -> [Spd], Trans Eta/2(SpdIn)
  EngTrq/1 -> Trans Eta/1(TrqIn), Product/2
  Diff Eta/1(eta) -> Divide2/1
  Divide2/1 -> EngTrqMaxWhls/1
  Divide3/1 -> Diff Eta/1(SpdIn)
  [Spd] -> Divide3/1

== system HevP1OptimalController/Series Regen Braking/MotTrq2WhlMotTrq/Diff Eta ==
  SpdIn : Inport
  TrqIn : Inport  Port=2
  Constant : Constant  Value=PlntDiffrntlEff
  Constant1 : Constant  SampleTime=-1
  Constant2 : Constant  Value=-1  SampleTime=-1
  Math Function1 : Math  Operator=pow  SignedPower=on  OutputSignalType=real
  Product1 : Product
  Switch2 : Switch  SaturateOnIntegerOverflow=off  InputSameDT=off
  rpm2rads : Gain  Gain=pi/30
  eta : Outport  VectorParamsAs1DForOutWhenUnconnected=off
  wires:
  rpm2rads/1 -> Product1/2
  Constant/1 -> Math Function1/1
  Constant2/1 -> Switch2/3
  Constant1/1 -> Switch2/1
  Product1/1 -> Switch2/2
  Switch2/1 -> Math Function1/2
  Math Function1/1 -> eta/1
  SpdIn/1 -> rpm2rads/1
  TrqIn/1 -> Product1/1

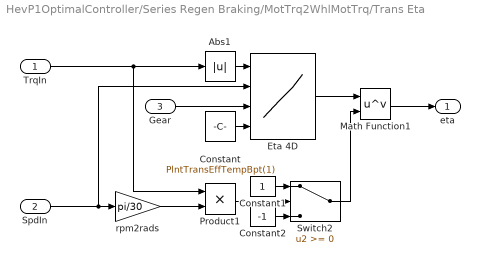
== system HevP1OptimalController/Series Regen Braking/MotTrq2WhlMotTrq/Trans Eta ==
  TrqIn : Inport
  SpdIn : Inport  Port=2
  Gear : Inport  Port=3
  Abs1 : Abs  SaturateOnIntegerOverflow=off
  Constant : Constant  Value=PlntTransEffTempBpt(1)
  Constant1 : Constant  SampleTime=-1
  Constant2 : Constant  Value=-1  SampleTime=-1
  Eta 4D : Lookup_n-D  NumberOfTableDimensions=4  LookupTableObject=''  BreakpointsForDimension1=PlntTransEffTrqBpt  BreakpointsForDimension2=PlntTransEffSpdBpt  BreakpointsForDimension3=PlntTransGearNumVect  BreakpointsForDimension4=PlntTransEffTempBpt  Table=PlntTransEffTbl  ExtrapMethod=Clip  InternalRulePriority=Speed  RndMeth=Simplest
      settings: InputPortMap=u0,u1,u2,u3
  Math Function1 : Math  Operator=pow  SignedPower=on  OutputSignalType=real
  Product1 : Product
  Switch2 : Switch  SaturateOnIntegerOverflow=off  InputSameDT=off
  rpm2rads : Gain  Gain=pi/30
  eta : Outport  VectorParamsAs1DForOutWhenUnconnected=off
  wires:
  TrqIn/1 -> Product1/1, Abs1/1
  SpdIn/1 -> Eta 4D/2, rpm2rads/1
  Math Function1/1 -> eta/1
  Abs1/1 -> Eta 4D/1
  Switch2/1 -> Math Function1/2
  Product1/1 -> Switch2/2
  Constant1/1 -> Switch2/1
  Constant2/1 -> Switch2/3
  Eta 4D/1 -> Math Function1/1
  rpm2rads/1 -> Product1/2
  Gear/1 -> Eta 4D/3
  Constant/1 -> Eta 4D/4

== system HevP1OptimalController/Series Regen Braking/EngBrakingEstimate/Transmission/Diff Eta ==
  note: Pwr >= 0, v = 1
      | Pwr < 0, v= -1
  SpdIn : Inport
  TrqIn : Inport  Port=2
  Constant : Constant  Value=PlntDiffrntlEff
  Constant1 : Constant  SampleTime=-1
  Constant2 : Constant  Value=-1  SampleTime=-1
  Math Function1 : Math  Operator=pow  SignedPower=on  OutputSignalType=real
  Product1 : Product
  Switch2 : Switch  SaturateOnIntegerOverflow=off  InputSameDT=off
  rpm2rads : Gain  Gain=pi/30
  eta : Outport  VectorParamsAs1DForOutWhenUnconnected=off
  wires:
  rpm2rads/1 -> Product1/2
  Constant/1 -> Math Function1/1
  Constant2/1 -> Switch2/3
  Constant1/1 -> Switch2/1
  Product1/1 -> Switch2/2
  Switch2/1 -> Math Function1/2
  Math Function1/1 -> eta/1
  SpdIn/1 -> rpm2rads/1
  TrqIn/1 -> Product1/1

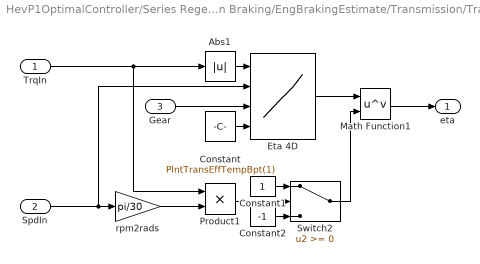
== system HevP1OptimalController/Series Regen Braking/EngBrakingEstimate/Transmission/Trans Eta ==
  TrqIn : Inport
  SpdIn : Inport  Port=2
  Gear : Inport  Port=3
  Abs1 : Abs  SaturateOnIntegerOverflow=off
  Constant : Constant  Value=PlntTransEffTempBpt(1)
  Constant1 : Constant  SampleTime=-1
  Constant2 : Constant  Value=-1  SampleTime=-1
  Eta 4D : Lookup_n-D  NumberOfTableDimensions=4  LookupTableObject=''  BreakpointsForDimension1=PlntTransEffTrqBpt  BreakpointsForDimension2=PlntTransEffSpdBpt  BreakpointsForDimension3=PlntTransGearNumVect  BreakpointsForDimension4=PlntTransEffTempBpt  Table=PlntTransEffTbl  ExtrapMethod=Clip  InternalRulePriority=Speed  RndMeth=Simplest
      settings: InputPortMap=u0,u1,u2,u3
  Math Function1 : Math  Operator=pow  SignedPower=on  OutputSignalType=real
  Product1 : Product
  Switch2 : Switch  SaturateOnIntegerOverflow=off  InputSameDT=off
  rpm2rads : Gain  Gain=pi/30
  eta : Outport  VectorParamsAs1DForOutWhenUnconnected=off
  wires:
  TrqIn/1 -> Product1/1, Abs1/1
  SpdIn/1 -> Eta 4D/2, rpm2rads/1
  Math Function1/1 -> eta/1
  Abs1/1 -> Eta 4D/1
  Switch2/1 -> Math Function1/2
  Product1/1 -> Switch2/2
  Constant1/1 -> Switch2/1
  Constant2/1 -> Switch2/3
  Eta 4D/1 -> Math Function1/1
  rpm2rads/1 -> Product1/2
  Gear/1 -> Eta 4D/3
  Constant/1 -> Eta 4D/4

== stateflow chart HevP1OptimalController/P2 Cltch1Cmd/P2 Cltch1Cmd/Chart ==
  state Unlocked
    du:
    Cltch1Cmd = 0;
  state Locked
    du:
    Cltch1Cmd = 1;
  (default) -> Unlocked
  Unlocked -> Locked : [EngTrqCmd > 0 && VehSpd > 1.8]
  Locked -> Unlocked : [VehSpd < 1.2]
  data: EngTrqCmd input; Cltch1Cmd output; VehSpd input
